simulink model "first"  (R2023a)
settings: Solver=VariableStepAuto  StartTime=0.0  StopTime=10.0  RelTol=1e-3
values from neighbouring files (symbols this model uses):
  Cm = 1.3    [constants.m]
  Comega = 3.15    [constants.m]
  Jdv = 7*10^(-6)    (= 7e-06)    [constants.m]
  Lov = 0.013    [constants.m]
  Lya = 0.0015    [constants.m]
  Rya = 8    [constants.m]
settings Model: Creator=Alla  LastModifiedBy=Alla

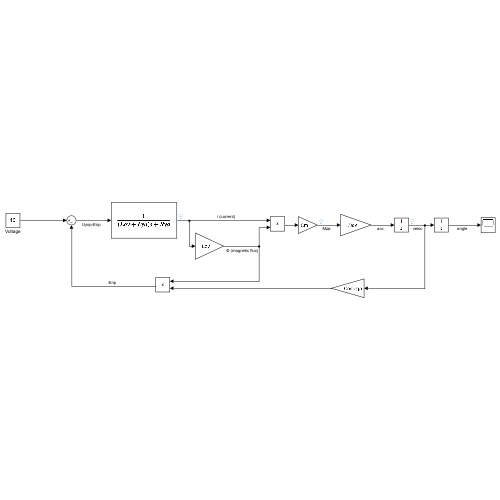
[thumbnail: Simulink's stored preview of the top-level diagram]
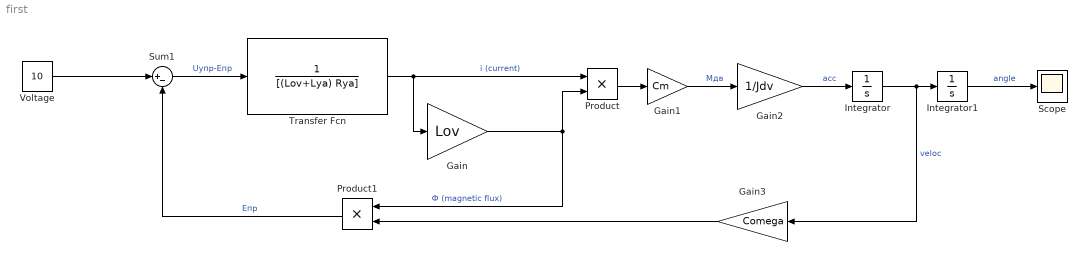
== system first ==
  Gain : Gain  Gain=Lov
  Gain1 : Gain  Gain=Cm
  Gain2 : Gain  Gain=1/Jdv
  Gain3 : Gain  Gain=Comega
  Integrator : Integrator
  Integrator1 : Integrator
  Product : Product
  Product1 : Product
  Scope : Scope
  Sum1 : Sum  Inputs=|+-
  Transfer Fcn : TransferFcn  Denominator=[(Lov+Lya) Rya]
  Voltage : Constant  Value=10
  wires:
  Voltage/1 -> Sum1/1
  Sum1/1 -> Transfer Fcn/1  "Uупр-Eпр"
  Transfer Fcn/1 -> Product/1, Gain/1  "i (current)"
  Gain/1 -> Product1/1, Product/2  "Ф (magnetic flux)"
  Product/1 -> Gain1/1
  Gain1/1 -> Gain2/1  "Mдв"
  Gain2/1 -> Integrator/1  "acc"
  Integrator/1 -> Integrator1/1, Gain3/1  "veloc"
  Integrator1/1 -> Scope/1  "angle"
  Gain3/1 -> Product1/2
  Product1/1 -> Sum1/2  "Eпр"
